simulink model "sampleModel2018"  (R2023a)
settings: Solver=VariableStepAuto  StartTime=0.0  StopTime=10.0  RelTol=1e-3
libraries: hdlsllib x10, simulink x1
settings Model: Creator=user1  LastModifiedBy=user1

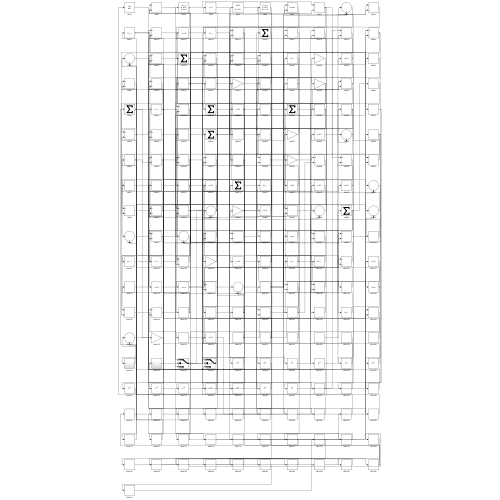
[thumbnail: Simulink's stored preview of the top-level diagram]
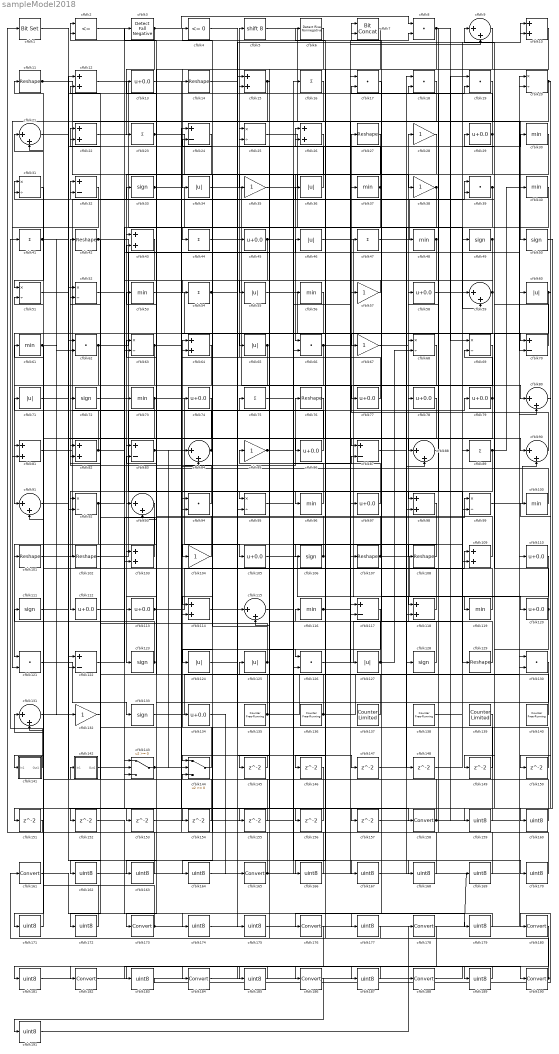
== system sampleModel2018 ==
  cfblk1 : simulink/Logic and Bit Operations/Bit Set  iBit=0
      settings: LibrarySourceBlock=|
      | hdlsllib/Logic and Bit
      | Operations/Bit Set
  cfblk{10,12,15,22,26,43,64,81..82,98,103,109,114,118} (14 alike) : Sum
  cfblk{30,37,40,48,53,56,61,73,96,100,116,119} (12 alike) : MinMax
  cfblk{11,14,27,42,76,101..102,107..108,129} (10 alike) : Reshape
  cfblk{28,35,38,57,67,85,104,132} (8 alike) : Gain
  cfblk{13,29,45,58,74,77..79,86,97,105,110,112..113,120,134} (16 alike) : Bias  Bias=0.0  SaturateOnIntegerOverflow=off
  cfblk{33,49..50,72,106,111,123,128,133} (9 alike) : Signum
  cfblk{9,21,59,80,84,88,90..91,93,115,131} (11 alike) : Sum  Inputs=|++
  cfblk{24,32,70,83,87,117,122} (7 alike) : Sum  Inputs=+-
  cfblk{8,17..19,39,62,66,94,121,126,130} (11 alike) : DotProduct  OutDataTypeStr=Inherit: Inherit via internal rule
  cfblk{34,36,46,55,60,65,71,124..125,127} (10 alike) : Abs  SaturateOnIntegerOverflow=off
  cfblk{135..136,138,140} (4 alike) : hdlsllib/Sources/Counter Free-Running  NumBits=16  tsamp=-1
  cfblk137 : hdlsllib/Sources/Counter Limited  uplimit=7  tsamp=-1
  cfblk139 : hdlsllib/Sources/Counter Limited  uplimit=7  tsamp=-1
  cfblk141 : Subsystem
      settings: LibrarySourceBlock=|
      | hdlsllib/Ports &
      | Subsystems/Subsystem
  cfblk142 : Subsystem
      settings: LibrarySourceBlock=|
      | hdlsllib/Ports &
      | Subsystems/Subsystem
  cfblk143 : Switch  SaturateOnIntegerOverflow=off  InputSameDT=off
  cfblk144 : Switch  SaturateOnIntegerOverflow=off  InputSameDT=off
  cfblk{145..157} (13 alike) : Delay  SampleTime=1
  cfblk{158,161,165,173,176,178,180,182,184,186,188,190} (12 alike) : DataTypeConversion  SaturateOnIntegerOverflow=off  RndMeth=Floor
  cfblk{159..160,162..164,166..172,174..175,177,179,181,183,185,187,189,191} (22 alike) : DataTypeConversion  OutDataTypeStr=uint8  SaturateOnIntegerOverflow=off  RndMeth=Floor
  cfblk{16,23,41,44,47,54,75,89} (8 alike) : Sum  Inputs=+
  cfblk2 : RelationalOperator  Operator=<=  OutDataTypeStr=boolean  InputSameDT=off
  cfblk{20,25,31,51..52,63,68..69,92,95,99} (11 alike) : Product  Inputs=*/  RndMeth=Zero  SaturateOnIntegerOverflow=on
  cfblk3 : hdlsllib/Logic and Bit Operations/Detect Fall Negative  vinit=0  OutDataTypeStr=boolean
  cfblk4 : hdlsllib/Logic and Bit Operations/Compare To Zero  relop=<=  OutDataTypeStr=boolean
  cfblk5 : ArithShift  BitShiftNumber=8
  cfblk6 : hdlsllib/Logic and Bit Operations/Detect Rise Nonnegative  vinit=0  OutDataTypeStr=boolean
  cfblk7 : hdlsllib/Logic and Bit Operations/Bit Concat  numInputs=2
  wires:
  cfblk129/1 -> cfblk28/1
  cfblk27/1 -> cfblk66/1
  cfblk59/1 -> cfblk91/1, cfblk54/1
  cfblk107/1 -> cfblk120/1, cfblk53/1
  cfblk89/1 -> cfblk112/1, cfblk40/1, cfblk166/1
  cfblk74/1 -> cfblk123/1
  cfblk5/1 -> cfblk50/1
  cfblk83/1 -> cfblk76/1, cfblk126/2
  cfblk66/1 -> cfblk118/1, cfblk103/2
  cfblk141/1(Out1) -> cfblk41/1
  cfblk144/1 -> cfblk64/1
  cfblk56/1 -> cfblk144/1
  cfblk139/1 -> cfblk142/1(In1)
  cfblk73/1 -> cfblk105/1, cfblk91/2, cfblk13/1
  cfblk93/1 -> cfblk121/1
  cfblk45/1 -> cfblk108/1, cfblk154/1
  cfblk12/1 -> cfblk44/1
  cfblk101/1 -> cfblk39/1
  cfblk104/1 -> cfblk94/1
  cfblk120/1 -> cfblk29/1, cfblk159/1
  cfblk49/1 -> cfblk124/1, cfblk126/1
  cfblk134/1 -> cfblk165/1
  cfblk123/1 -> cfblk11/1, cfblk32/2
  cfblk143/1 -> cfblk46/1, cfblk84/1, cfblk78/1
  cfblk78/1 -> cfblk88/1
  cfblk82/1 -> cfblk42/1, cfblk48/1
  cfblk137/1 -> cfblk75/1
  cfblk114/1 -> cfblk115/1
  cfblk26/1 -> cfblk94/2
  cfblk121/1 -> cfblk133/1
  cfblk118/1 -> cfblk74/1
  cfblk130/1 -> cfblk173/1
  cfblk105/1 -> cfblk119/1
  cfblk77/1 -> cfblk5/1
  cfblk46/1 -> cfblk80/1
  cfblk33/1 -> cfblk128/1, cfblk84/2
  cfblk102/1 -> cfblk79/1
  cfblk108/1 -> cfblk104/1
  cfblk62/1 -> cfblk81/1, cfblk20/2
  cfblk96/1 -> cfblk85/1
  cfblk7/1 -> cfblk34/1
  cfblk25/1 -> cfblk117/1
  cfblk10/1 -> cfblk106/1
  cfblk116/1 -> cfblk109/1, cfblk8/2, cfblk9/2
  cfblk60/1 -> cfblk149/1, cfblk150/1
  cfblk128/1 -> cfblk7/1
  cfblk28/1 -> cfblk93/1
  cfblk138/1 -> cfblk89/1
  cfblk51/1 -> cfblk12/1
  cfblk126/1 -> cfblk59/1
  cfblk24/1 -> cfblk43/1
  cfblk125/1 -> cfblk32/1, cfblk24/2
  cfblk35/1 -> cfblk38/1
  cfblk42/1 -> cfblk90/1, cfblk172/1
  cfblk55/1 -> cfblk127/1
  cfblk48/1 -> cfblk95/1, cfblk73/1
  cfblk41/1 -> cfblk30/1, cfblk132/1
  cfblk86/1 -> cfblk4/1
  cfblk3/1 -> cfblk8/1, cfblk23/1
  cfblk31/1 -> cfblk51/1
  cfblk133/1 -> cfblk60/1
  cfblk40/1 -> cfblk86/1
  cfblk19/1 -> cfblk117/2
  cfblk36/1 -> cfblk15/2
  cfblk90/1 -> cfblk27/1
  cfblk140/1 -> cfblk125/1
  cfblk75/1 -> cfblk57/1
  cfblk72/1 -> cfblk129/1
  cfblk34/1 -> cfblk77/1
  cfblk32/1 -> cfblk81/2
  cfblk69/1 -> cfblk87/1
  cfblk99/1 -> cfblk90/2
  cfblk8/1 -> cfblk98/1, cfblk69/1, cfblk93/2
  cfblk18/1 -> cfblk113/1
  cfblk29/1 -> cfblk35/1, cfblk17/2
  cfblk22/1 -> cfblk59/2
  cfblk124/1 -> cfblk10/1
  cfblk115/1 -> cfblk87/2
  cfblk76/1 -> cfblk141/1(In1)
  cfblk106/1 -> cfblk2/1, cfblk83/2
  cfblk1/1 -> cfblk122/2
  cfblk65/1 -> cfblk64/2, cfblk114/2
  cfblk100/1 -> cfblk33/1
  cfblk79/1 -> cfblk69/2, cfblk162/1
  cfblk84/1 -> cfblk51/2, cfblk22/2
  cfblk39/1 -> cfblk98/2, cfblk9/1
  cfblk47/1 -> cfblk39/2
  cfblk52/1 -> cfblk158/1
  cfblk119/1 -> cfblk71/1
  cfblk37/1 -> cfblk6/1, cfblk63/2
  cfblk94/1 -> cfblk72/1
  cfblk63/1 -> cfblk92/1, cfblk156/1
  cfblk136/1 -> cfblk88/2, cfblk26/2, cfblk82/1, cfblk63/1
  cfblk97/1 -> cfblk36/1
  cfblk20/1 -> cfblk96/1, cfblk160/1
  cfblk95/1 -> cfblk109/2
  cfblk81/1 -> cfblk3/1
  cfblk135/1 -> cfblk80/2, cfblk82/2
  cfblk122/1 -> cfblk99/1
  cfblk61/1 -> cfblk62/2, cfblk171/1
  cfblk38/1 -> cfblk67/1, cfblk114/1
  cfblk58/1 -> cfblk10/2
  cfblk127/1 -> cfblk43/2, cfblk68/2
  cfblk113/1 -> cfblk97/1, cfblk49/1
  cfblk15/1 -> cfblk115/2, cfblk121/2
  cfblk67/1 -> cfblk68/1
  cfblk11/1 -> cfblk56/1, cfblk70/2
  cfblk57/1 -> cfblk55/1
  cfblk2/1 -> cfblk7/2
  cfblk109/1 -> cfblk2/2
  cfblk53/1 -> cfblk65/1
  cfblk111/1 -> cfblk19/2
  cfblk112/1 -> cfblk143/1
  cfblk142/1(Out1) -> cfblk143/2
  cfblk43/1 -> cfblk143/3
  cfblk9/1 -> cfblk14/1
  cfblk71/1 -> cfblk83/1
  cfblk4/1 -> cfblk95/2
  cfblk80/1 -> cfblk100/1
  cfblk85/1 -> cfblk37/1, cfblk168/1
  cfblk13/1 -> cfblk70/1
  cfblk92/1 -> cfblk25/1, cfblk101/1
  cfblk68/1 -> cfblk102/1
  cfblk23/1 -> cfblk103/1, cfblk47/1
  cfblk64/1 -> cfblk92/2
  cfblk54/1 -> cfblk45/1, cfblk26/1
  cfblk103/1 -> cfblk22/1
  cfblk70/1 -> cfblk31/1
  cfblk88/1 -> cfblk58/1
  cfblk117/1 -> cfblk145/1
  cfblk145/1 -> cfblk144/2
  cfblk98/1 -> cfblk146/1
  cfblk146/1 -> cfblk144/3
  cfblk14/1 -> cfblk147/1
  cfblk147/1 -> cfblk118/2
  cfblk87/1 -> cfblk148/1
  cfblk148/1 -> cfblk99/2
  cfblk149/1 -> cfblk15/1
  cfblk150/1 -> cfblk12/2
  cfblk50/1 -> cfblk151/1
  cfblk151/1 -> cfblk1/1
  cfblk132/1 -> cfblk152/1
  cfblk91/1 -> cfblk153/1
  cfblk153/1 -> cfblk66/2
  cfblk154/1 -> cfblk122/1
  cfblk6/1 -> cfblk155/1
  cfblk155/1 -> cfblk62/1
  cfblk156/1 -> cfblk31/2
  cfblk17/1 -> cfblk157/1
  cfblk157/1 -> cfblk20/1
  cfblk158/1 -> cfblk17/1, cfblk19/1
  cfblk159/1 -> cfblk52/1
  cfblk160/1 -> cfblk52/2
  cfblk162/1 -> cfblk110/1
  cfblk16/1 -> cfblk163/1
  cfblk163/1 -> cfblk111/1
  cfblk30/1 -> cfblk164/1
  cfblk164/1 -> cfblk16/1
  cfblk165/1 -> cfblk24/1, cfblk107/1
  cfblk166/1 -> cfblk134/1
  cfblk21/1 -> cfblk167/1
  cfblk167/1 -> cfblk18/1
  cfblk168/1 -> cfblk21/1
  cfblk169/1 -> cfblk21/2
  cfblk131/1 -> cfblk170/1
  cfblk170/1 -> cfblk18/2
  cfblk171/1 -> cfblk131/1
  cfblk172/1 -> cfblk131/2
  cfblk173/1 -> cfblk169/1, cfblk61/1
  cfblk152/1 -> cfblk174/1
  cfblk174/1 -> cfblk130/1
  cfblk44/1 -> cfblk175/1
  cfblk175/1 -> cfblk130/2
  cfblk110/1 -> cfblk177/1
  cfblk177/1 -> cfblk161/1
  cfblk161/1 -> cfblk179/1
  cfblk179/1 -> cfblk176/1
  cfblk176/1 -> cfblk181/1
  cfblk181/1 -> cfblk178/1
  cfblk178/1 -> cfblk183/1
  cfblk183/1 -> cfblk180/1
  cfblk180/1 -> cfblk185/1
  cfblk185/1 -> cfblk182/1
  cfblk182/1 -> cfblk187/1
  cfblk187/1 -> cfblk184/1
  cfblk188/1 -> cfblk190/1
  cfblk184/1 -> cfblk189/1
  cfblk189/1 -> cfblk186/1
  cfblk190/1 -> cfblk25/2, cfblk116/1
  cfblk186/1 -> cfblk191/1
  cfblk191/1 -> cfblk188/1

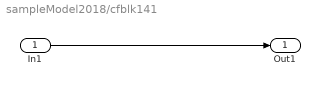
== system sampleModel2018/cfblk141 ==
  In1 : Inport
  Out1 : Outport
  wires:
  In1/1 -> Out1/1

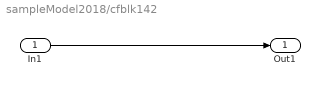
== system sampleModel2018/cfblk142 ==
  In1 : Inport
  Out1 : Outport
  wires:
  In1/1 -> Out1/1
